simulink library "libMdl_invQuat"  (R2018a)
settings: Solver=VariableStepAuto  StartTime=0.0  StopTime=10.0  RelTol=1e-3
settings Model: Creator=hwinter  LastModifiedBy=Hanno

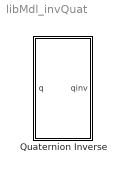
== system libMdl_invQuat ==
  Quaternion Inverse : Subsystem
      mask Display:
      | color('black')
      | port_label('input', 1, 'q', 'texmode','on')
      | port_label('output', 1, 'q^{-1}', 'texmode','on')

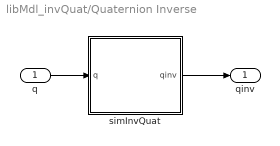
== system libMdl_invQuat/Quaternion Inverse ==
  q : Inport
  simInvQuat : MATLAB Function  TreatAsAtomicUnit=on
  qinv : Outport
  wires:
  q/1 -> simInvQuat/1(q)
  simInvQuat/1(qinv) -> qinv/1

== matlab function libMdl_invQuat/Quaternion Inverse/simInvQuat ==
  data: q input; qinv output
function qinv = simInvQuat(q)

qinv = invQuat(q);

end % function
